simulink model "zaj8simulink"  (R2020b)
settings: Solver=VariableStepAuto  StartTime=0.0  StopTime=2000.0  MaxStep=0.1  MinStep=0.01  RelTol=1e-3
values from neighbouring files (symbols this model uses):
  cv1 = ro*cp*v1    (= 108540)    [zaj1.m]
  cv2 = ro*cp*v2    (= 36180)    [zaj1.m]
  dqg = 1000    [zaj1.m]
  dT2N = 5    [zaj1.m]
  dTzew = 0    [zaj1.m]
  k = 1.75/dqg    (= 0.00175)    [zaj1.m]
  Kp_chien0 = (0.35*T)/(k*T_0)*4.49    (= 26940)    [zaj1.m]
  Kp_chien20 = (0.6*T)/(k*T_0)    (= 10285.7142857)    [zaj1.m]
  Kp_nichols = (0.9*T)/(k*T_0)    (= 15428.5714286)    [zaj1.m]
  Ks0 = (Ks2*(T2N-TzewN))/(T1N-T2N)    (= 903.225806452)    [zaj1.m]
  Ks1 = 3*Ks2    (= 387.096774194)    [zaj1.m]
  Ks2 = QgN/(3*(T1N-TzewN)+T2N-TzewN)    (= 129.032258065)    [zaj1.m]
  QgN = 20000    [zaj1.m]
  steptime = 100    [zaj1.m]
  T = 300    [zaj1.m]
  T1N = 20    [zaj1.m]
  T2N = 15    [zaj1.m]
  T_0 = 10    [zaj1.m]
  Ti_chien0 = 1.2*T    (= 360)    [zaj1.m]
  Ti_chien20 = T    (= 300)    [zaj1.m]
  Ti_nichols = 3.33*T_0    (= 33.3)    [zaj1.m]
  tw10d = [cv1*cv2 cv1*Ks0+cv1*Ks2+Ks1*cv2+Ks0*cv2 Ks0*Ks1+Ks2*Ks0+Ks1*Ks2]    [zaj1.m]
  tw1intinit = T1N    (= 20)    [zaj1.m]
  tw2intinit = T2N    (= 15)    [zaj1.m]
  TzewN = -20    [zaj1.m]
settings Model: Creator=bilin  LastModifiedBy=bilin

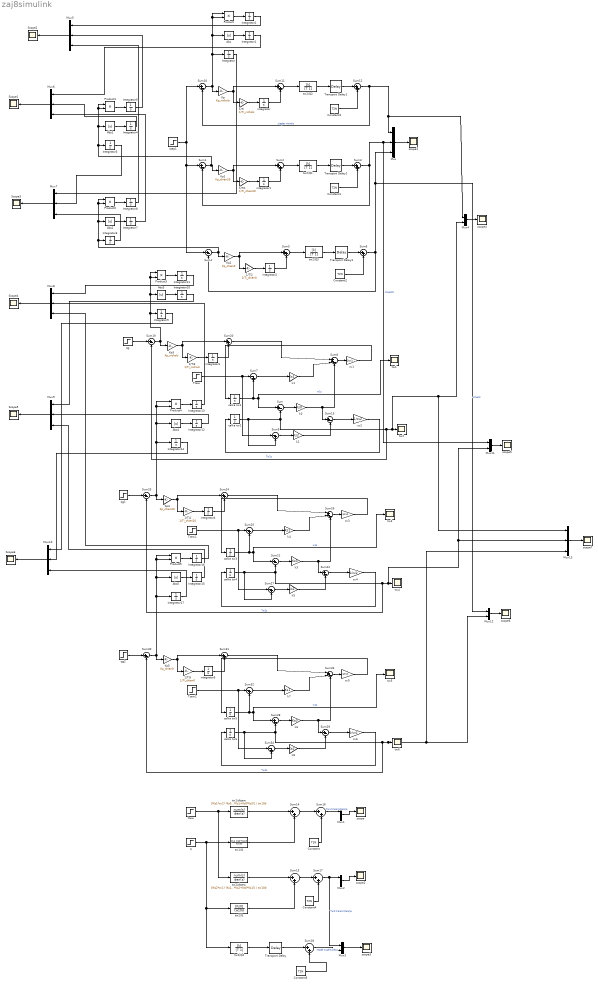
== system zaj8simulink ==
  1/Ti : Gain  Gain=1/Ti_nichols
  1/Ti1 : Gain  Gain=1/Ti_chien20
  1/Ti2 : Gain  Gain=1/Ti_chien0
  1/Ti3 : Gain  Gain=1/Ti_nichols
  1/Ti4 : Gain  Gain=1/Ti_chien20
  1/Ti5 : Gain  Gain=1/Ti_chien0
  Abs{,1..5} (6 alike) : Abs
  Constant : Constant  Value=T1N
  Constant{1..5} (5 alike) : Constant  Value=T2N
  Integrator{,1..17} (18 alike) : Integrator
  Kp : Gain  Gain=Kp_nichols
  Kp1 : Gain  Gain=Kp_chien20
  Kp2 : Gain  Gain=Kp_chien0
  Kp3 : Gain  Gain=Kp_nichols
  Kp4 : Gain  Gain=Kp_chien20
  Kp5 : Gain  Gain=Kp_chien0
  Mux{,5..10,13} (8 alike) : Mux  Inputs=3
  Mux{1..4,11..12} (6 alike) : Mux  Inputs=2
  Product{,1..5} (6 alike) : Product
  Scope{1..6} (6 alike) : Scope
  Sum{,1,4,10,13,19,21..23,28..30} (12 alike) : Sum  Inputs=|+-
  Sum{2..3,5..6,11..12,14..18,20,24,31} (14 alike) : Sum  Inputs=|++
  Sum{7,9,25,27,32,34} (6 alike) : Sum  Inputs=|-+
  Sum26 : Sum  Inputs=|+--
  Sum33 : Sum  Inputs=|+--
  Sum8 : Sum  Inputs=|+--
  Transport Delay{,1..3} (4 alike) : TransportDelay  DelayTime=T_0
  Tzew : Step  Time=100  Before=TzewN  After=TzewN+dTzew  SampleTime=0
  Tzew1 : Step  Time=100  Before=TzewN  After=TzewN+dTzew  SampleTime=0
  Tzew2 : Step  Time=100  Before=TzewN  After=TzewN+dTzew  SampleTime=0
  calka tw1 : Integrator  InitialCondition=tw1intinit
  calka tw2 : Integrator  InitialCondition=tw2intinit
  calka tw3 : Integrator  InitialCondition=tw1intinit
  calka tw4 : Integrator  InitialCondition=tw2intinit
  calka tw5 : Integrator  InitialCondition=tw1intinit
  calka tw6 : Integrator  InitialCondition=tw2intinit
  cv1 : Gain  Gain=1/cv1
  cv2 : Gain  Gain=1/cv2
  cv3 : Gain  Gain=1/cv1
  cv4 : Gain  Gain=1/cv2
  cv5 : Gain  Gain=1/cv1
  cv6 : Gain  Gain=1/cv2
  integrator : Integrator
  integrator1 : Integrator
  integrator2 : Integrator
  integrator3 : Integrator  InitialCondition=QgN
  integrator4 : Integrator  InitialCondition=QgN
  integrator5 : Integrator  InitialCondition=QgN
  k0 : Gain  Gain=Ks0
  k1 : Gain  Gain=Ks1
  k2 : Gain  Gain=Ks2
  k3 : Gain  Gain=Ks0
  k4 : Gain  Gain=Ks1
  k5 : Gain  Gain=Ks2
  k6 : Gain  Gain=Ks0
  k7 : Gain  Gain=Ks1
  k8 : Gain  Gain=Ks2
  q : Step  Time=steptime  After=dqg  SampleTime=0
  qg : Step  Time=100  Before=T2N  After=T2N+dT2N  SampleTime=0
  qg1 : Step  Time=100  Before=T2N  After=T2N+dT2N  SampleTime=0
  qg2 : Step  Time=100  Before=T2N  After=T2N+dT2N  SampleTime=0
  scope{,1..7} (8 alike) : Scope
  step1 : Step  Time=100  Before=T2N  After=T2N+dT2N  SampleTime=0
  tw{1..6} (6 alike) : Scope
  tw1/Q : TransferFcn  Numerator=[cv2 (Ks0+Ks2)]  Denominator=tw10d
  tw1/dtzew : TransferFcn  Numerator=[(Ks1*cv2) (Ks0*Ks1+Ks2*Ks1+Ks0*Ks2)]  Denominator=tw10d
  tw2/Q : TransferFcn  Numerator=[Ks0]  Denominator=tw10d
  tw2/Q{1..4} (4 alike) : TransferFcn  Numerator=[k]  Denominator=[T 1]
  tw2/dtzew : TransferFcn  Numerator=[(Ks2*cv1) (Ks1*Ks2+Ks0*Ks2+Ks0*Ks1)]  Denominator=tw10d
  tzew : Step  Time=steptime  After=dTzew  SampleTime=0
  wires:
  Sum12/1 -> Sum10/2, Mux/1, Mux4/1  "ziegler nichols"
  1/Ti/1 -> integrator/1
  Kp/1 -> Sum11/1, 1/Ti/1
  tw2/Q2/1 -> Transport Delay1/1
  Transport Delay1/1 -> Sum12/1
  integrator/1 -> Sum11/2
  Constant3/1 -> Sum12/2
  Sum10/1 -> Product/1, Product/2, Abs/1, Integrator/1, Kp/1
  Sum11/1 -> tw2/Q2/1
  Constant1/1 -> Sum3/2
  Sum2/1 -> tw2/Q1/1
  step1/1 -> Sum4/1, Sum1/1, Sum10/1
  Sum1/1 -> Product1/2, Product1/1, Abs1/1, Integrator3/1, Kp1/1
  integrator1/1 -> Sum2/2
  Transport Delay2/1 -> Sum3/1
  tw2/Q1/1 -> Transport Delay2/1
  Kp1/1 -> Sum2/1, 1/Ti1/1
  Sum3/1 -> Sum1/2, Mux11/1, Mux/2  "chien20"
  1/Ti1/1 -> integrator1/1
  Constant2/1 -> Sum6/2
  Sum5/1 -> tw2/Q3/1
  Sum4/1 -> Product2/2, Product2/1, Abs2/1, Integrator6/1, Kp2/1
  integrator2/1 -> Sum5/2
  Transport Delay3/1 -> Sum6/1
  tw2/Q3/1 -> Transport Delay3/1
  Kp2/1 -> Sum5/1, 1/Ti2/1
  Sum6/1 -> Sum4/2, Mux12/1, Mux/3  "chien0"
  1/Ti2/1 -> integrator2/1
  Mux/1 -> scope1/1
  Abs/1 -> Integrator1/1
  Product/1 -> Integrator2/1
  tw2/Q/1 -> Sum15/2
  Transport Delay/1 -> Sum18/1
  Sum14/1 -> Sum16/1
  Sum18/1 -> Mux3/2  "Model Kupfmullera"
  Constant/1 -> Sum16/2
  Constant5/1 -> Sum18/2
  Sum17/1 -> Mux2/1, Mux3/1  "Tw2 transmitancja"
  Mux1/1 -> scope/1
  tw1/dtzew/1 -> Sum14/1
  Mux3/1 -> scope3/1
  Constant4/1 -> Sum17/2
  q/1 -> tw2/Q/1, tw2/Q4/1, tw1/Q/1
  tw2/dtzew/1 -> Sum15/1
  Sum15/1 -> Sum17/1
  tw2/Q4/1 -> Transport Delay/1
  tw1/Q/1 -> Sum14/2
  Sum16/1 -> Mux1/1  "Tw1 transmitancja"
  tzew/1 -> tw2/dtzew/1, tw1/dtzew/1
  Mux2/1 -> scope2/1
  k0/1 -> Sum13/1, Sum8/3
  Sum7/1 -> k1/1
  cv2/1 -> calka tw2/1
  Sum8/1 -> cv1/1
  calka tw2/1 -> Sum9/2, Mux13/1, Mux4/2, tw2/1, Sum19/2, Sum/2  "Tw2s"
  k1/1 -> Sum8/2
  Sum13/1 -> cv2/1
  cv1/1 -> calka tw1/1
  Sum9/1 -> k2/1
  Tzew/1 -> Sum9/1, Sum7/1
  calka tw1/1 -> Sum7/2, tw1/1, Sum/1  "w1s"
  Sum/1 -> k0/1
  k2/1 -> Sum13/2
  Kp3/1 -> Sum20/1, 1/Ti3/1
  Sum19/1 -> Kp3/1, Product3/1, Product3/2, Abs3/1, Integrator9/1
  integrator3/1 -> Sum20/2
  1/Ti3/1 -> integrator3/1
  qg/1 -> Sum19/1
  Sum20/1 -> Sum8/1
  Mux4/1 -> scope4/1
  k3/1 -> Sum22/1, Sum26/3
  k5/1 -> Sum22/2
  Kp4/1 -> Sum24/1, 1/Ti4/1
  calka tw3/1 -> Sum25/2, tw3/1, Sum21/1  "w1s"
  Sum21/1 -> k3/1
  Tzew1/1 -> Sum27/1, Sum25/1
  integrator4/1 -> Sum24/2
  cv4/1 -> calka tw4/1
  Sum26/1 -> cv3/1
  Sum25/1 -> k4/1
  Sum22/1 -> cv4/1
  Sum23/1 -> Kp4/1, Product4/1, Product4/2, Abs4/1, Integrator14/1
  cv3/1 -> calka tw3/1
  Sum27/1 -> k5/1
  k4/1 -> Sum26/2
  1/Ti4/1 -> integrator4/1
  calka tw4/1 -> Sum27/2, Mux13/2, Mux11/2, tw4/1, Sum23/2, Sum21/2  "Tw2s"
  Sum24/1 -> Sum26/1
  qg1/1 -> Sum23/1
  k6/1 -> Sum29/1, Sum33/3
  k8/1 -> Sum29/2
  Kp5/1 -> Sum31/1, 1/Ti5/1
  calka tw5/1 -> Sum32/2, tw5/1, Sum28/1  "w1s"
  Sum28/1 -> k6/1
  Tzew2/1 -> Sum34/1, Sum32/1
  integrator5/1 -> Sum31/2
  cv6/1 -> calka tw6/1
  Sum33/1 -> cv5/1
  Sum32/1 -> k7/1
  Sum29/1 -> cv6/1
  Sum30/1 -> Kp5/1, Product5/1, Product5/2, Abs5/1, Integrator17/1
  cv5/1 -> calka tw5/1
  Sum34/1 -> k8/1
  k7/1 -> Sum33/2
  1/Ti5/1 -> integrator5/1
  calka tw6/1 -> Sum34/2, Mux13/3, Mux12/2, tw6/1, Sum30/2, Sum28/2  "Tw2s"
  Sum31/1 -> Sum33/1
  qg2/1 -> Sum30/1
  Product1/1 -> Integrator5/1
  Abs1/1 -> Integrator4/1
  Abs2/1 -> Integrator7/1
  Product2/1 -> Integrator8/1
  Product3/1 -> Integrator11/1
  Abs3/1 -> Integrator10/1
  Abs4/1 -> Integrator12/1
  Product4/1 -> Integrator13/1
  Product5/1 -> Integrator16/1
  Abs5/1 -> Integrator15/1
  Mux5/1 -> Scope2/1
  Mux6/1 -> Scope1/1
  Mux7/1 -> Scope3/1
  Integrator2/1 -> Mux5/1
  Integrator5/1 -> Mux5/2
  Integrator8/1 -> Mux5/3
  Integrator1/1 -> Mux6/1
  Integrator4/1 -> Mux6/2
  Integrator/1 -> Mux7/1
  Integrator3/1 -> Mux7/2
  Integrator6/1 -> Mux7/3
  Integrator7/1 -> Mux6/3
  Mux8/1 -> Scope4/1
  Mux9/1 -> Scope5/1
  Mux10/1 -> Scope6/1
  Integrator11/1 -> Mux8/1
  Integrator13/1 -> Mux8/2
  Integrator16/1 -> Mux8/3
  Integrator10/1 -> Mux9/1
  Integrator12/1 -> Mux9/2
  Integrator15/1 -> Mux9/3
  Integrator9/1 -> Mux10/1
  Integrator14/1 -> Mux10/2
  Integrator17/1 -> Mux10/3
  Mux11/1 -> scope5/1
  Mux12/1 -> scope6/1
  Mux13/1 -> scope7/1
